simulink model "sas"  (R2018a)
settings: Solver=VariableStepAuto  StartTime=0.0  StopTime=10.0  RelTol=1e-3
values from neighbouring files (symbols this model uses):
  A = [-0.019311 -0.00025389 0 2.9465e-12 0 0 8.8157 -1.0189 0 0.82225 0 10 ... (36 elements, 6x6)]    [ABCD.mat]
  B = [0 0 0 0 20.2 0]    [ABCD.mat]
  C = [0 0 0 57.2957795131 0 0 0 0 0 0 57.2957795131 0 ... (18 elements, 3x6)]    [ABCD.mat]
  D = [0 0 0]    [ABCD.mat]
settings Model: Creator=user  LastModifiedBy=user

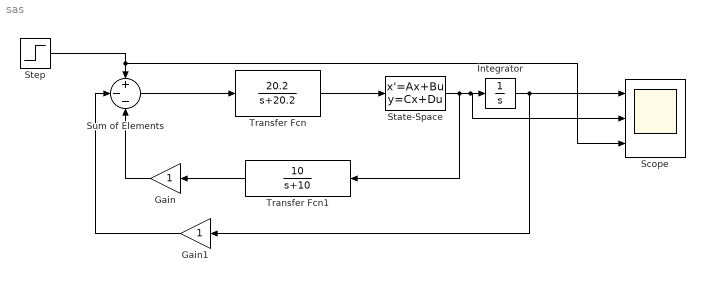
== system sas ==
  Gain : Gain
  Gain1 : Gain
  Integrator : Integrator
  Scope : Scope  NumInputPorts=3
  State-Space : StateSpace  A=A  B=B  C=C  D=D  InitialCondition=0
  Step : Step  SampleTime=0
  Sum of Elements : Sum  Inputs=+--
  Transfer Fcn : TransferFcn  Numerator=[20.2]  Denominator=[1 20.2]
  Transfer Fcn1 : TransferFcn  Numerator=[10]  Denominator=[1 10]
  wires:
  Transfer Fcn/1 -> State-Space/1
  Sum of Elements/1 -> Transfer Fcn/1
  State-Space/1 -> Integrator/1, Scope/2, Transfer Fcn1/1
  Transfer Fcn1/1 -> Gain/1
  Integrator/1 -> Gain1/1, Scope/1
  Step/1 -> Scope/3, Sum of Elements/1
  Gain/1 -> Sum of Elements/3
  Gain1/1 -> Sum of Elements/2
